simulink model "part3model"  (R2021b)
settings: Solver=VariableStepAuto  StartTime=0.0  StopTime=10.0  RelTol=1e-3
libraries: spsDiodeLib x6, spsVoltageMeasurementLib x2, spsACCurrentSourceLib x1, spsGroundLib x1, spsThreePhaseSourceLib x1, spspowerguiLib x1
settings Model: Creator=ardak  LastModifiedBy=ardak

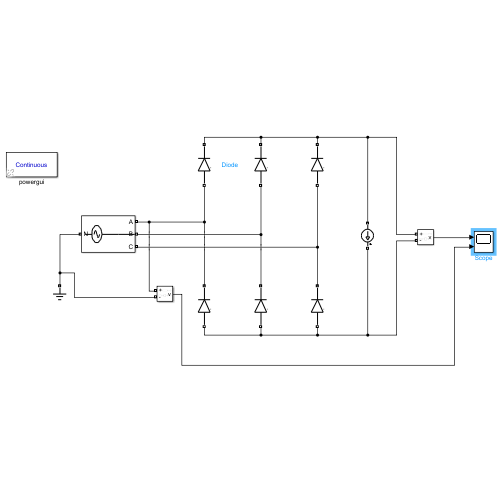
[thumbnail: Simulink's stored preview of the top-level diagram]
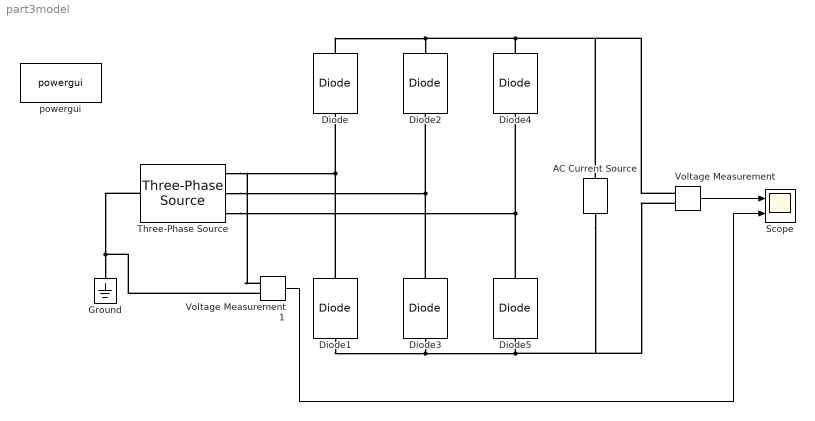
== system part3model ==
  AC Current Source : spsACCurrentSourceLib/AC Current Source  Amplitude=60  Phase=90  Frequency=0  SampleTime=0  Measurements=None
      settings: SourceProductBaseCode=PS
  Diode{,1..5} (6 alike) : spsDiodeLib/Diode  Ron=0.001  Lon=0  Vf=0.8  IC=0  UseSnubber=0  Rs=inf  Cs=0  Measurements=off
  Ground : spsGroundLib/Ground  LConnTagsString=a
  Scope : Scope  NumInputPorts=2
  Three-Phase Source : spsThreePhaseSourceLib/Three-Phase Source  InternalConnection=Yn  VoltagePhases=off  Voltage=400  PhaseAngle=0  Voltage_phases=[400 400 400]/sqrt(3)  PhaseAngles_phases=[0 -120 +120]  Frequency=50  NonIdealSource=off  SpecifyImpedance=off  Resistance=0  Inductance=0  ShortCircuitLevel=100e6  BaseVoltage=400  XRratio=7  BusType=swing  Pref=10e3  Qref=0  Prefabc=[10e3, 10e3, 10e3]  Qrefabc=[0, 0, 0]  Qmin=-inf  Qmax=inf
  Voltage Measurement : spsVoltageMeasurementLib/Voltage Measurement  PhasorSimulation=off  OutputType=Complex  PSBequivalent=0
  Voltage Measurement1 : spsVoltageMeasurementLib/Voltage Measurement  PhasorSimulation=off  OutputType=Complex  PSBequivalent=0
  powergui : spspowerguiLib/powergui  Priority=1  SimulationMode=Continuous  SampleTime=50e-6  frequency=60  Iterations=50  frequencyindice=50  Pbase=100e6  ErrMax=1e-4  UnitsV=kV  UnitsW=MW  buscounter=0  FunctionMessages=off  echomessages=off  EnableUseOfTLC=off  CurrentSourceSwitches=off  DisableSnubberDevices=off  DisableRonSwitches=off  DisableVfSwitches=off  DisplayEquations=off  AutomaticDiscreteSolvers=off  SolverType=Tustin/Backward Euler (TBE)  Interpol=off  ExternalGateDelay=off  methode=off  Ts=100  x0status=blocks  SPID=on  SwTol=0  HookPort=off  NonlinearTolerance=1e-4  nMaxIteration=100  ContinueOnMaxIteration=off  RestoreLinks=warning  ResistiveCurrentMeasurement=off  Frange=[0:2:500]  Ylog=off  Xlog=on  ShowGrid=off  save=off  variable=ZData  structure=0  ZoomFFT=off  StartTime=0.0  cycles=1  DisplayStyle=1  fundamental=60  FreqAxis=off  MaxFrequency=1000  frequencyindicesteady=1  RmsSteady=1  display=off
  wires:
  Voltage Measurement/1 -> Scope/1
  Voltage Measurement1/1 -> Scope/2
  connections:
  Diode1/RConn1 -- Voltage Measurement1/LConn1 -- Three-Phase Source/RConn1 -- Diode/LConn1
  Diode3/RConn1 -- Three-Phase Source/RConn2 -- Diode2/LConn1
  Diode5/RConn1 -- Three-Phase Source/RConn3 -- Diode4/LConn1
  Diode/RConn1 -- AC Current Source/LConn1 -- Voltage Measurement/LConn1 -- Diode4/RConn1 -- Diode2/RConn1
  Diode1/LConn1 -- Diode3/LConn1 -- AC Current Source/RConn1 -- Voltage Measurement/LConn2 -- Diode5/LConn1
  Voltage Measurement1/LConn2 -- Three-Phase Source/LConn1 -- Ground/LConn1
